simulink model "Sim_PS_DynamicOBS"  (R2018b)
settings: Solver=FixedStepAuto  StartTime=0.0  StopTime=sim_time  FixedStep=Ts  RelTol=1e-3
values from neighbouring files (symbols this model uses):
  obs1 = [x_obs1;y_obs1;r_obs1]    [Main_dynamic_obs.m]    (also in Main_static_obs.m)
  Ref = [1;1;0]    [Main_dynamic_obs.m]    (also in Main_static_obs.m)
  th0 = 0    [Main_dynamic_obs.m]    (also in Main_static_obs.m)
  Ts = 0.1    [Main_dynamic_obs.m]    (also in Main_static_obs.m)
  x0 = -1    [Main_dynamic_obs.m]    (also in Main_static_obs.m)
  x_obs2 = -0.25    [Main_dynamic_obs.m]    (also in Main_static_obs.m = 0.5)
  y0 = -1    [Main_dynamic_obs.m]    (also in Main_static_obs.m)
  y_obs2 = -0.25    [Main_dynamic_obs.m]    (also in Main_static_obs.m = 0.5)
libraries: simulink x1
settings Model: Creator=sanim  LastModifiedBy=sanim

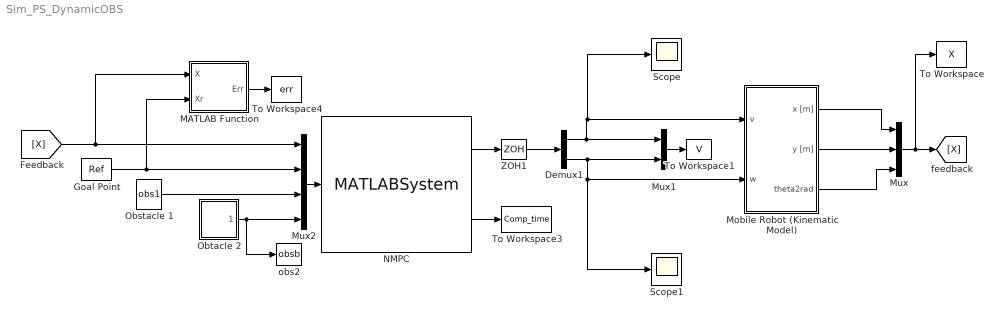
== system Sim_PS_DynamicOBS ==
  Demux1 : Demux  Outputs=2
  Goal Point : Constant  Value=Ref  SampleTime=Ts
  MATLAB Function : MATLAB Function  TreatAsAtomicUnit=on
  Mobile Robot (Kinematic Model) : Subsystem
  Mux : Mux  Inputs=3
  Mux1 : Mux  Inputs=2
  Mux2 : Mux
  NMPC : MATLABSystem  System=single_robot_obs  SimulateUsing=Interpreted execution
      mask Type: single_robot_obs
      mask Display:
      | disp('single_robot_obs');
      | port_label('input',1,'x');
      | port_label('output',1,'u');
      | port_label('output',2,'comp_time');
  Obstacle 1 : Constant  Value=obs1  SampleTime=Ts
  Obtacle 2 : Subsystem
  Scope : Scope
  Scope1 : Scope
  To Workspace : ToWorkspace  VariableName=X  SaveFormat=Structure With Time  SampleTime=Ts
  To Workspace1 : ToWorkspace  VariableName=V  SaveFormat=Structure With Time  SampleTime=Ts
  To Workspace3 : ToWorkspace  VariableName=Comp_time  SaveFormat=Structure  SampleTime=Ts
      settings: Save2DSignal=2-D array (concatenate along first dimension)
  To Workspace4 : ToWorkspace  VariableName=err  SampleTime=Ts
      settings: Save2DSignal=2-D array (concatenate along first dimension)
  ZOH1 : ZeroOrderHold  SampleTime=Ts
  obs2 : ToWorkspace  VariableName=obsb  SaveFormat=Structure  SampleTime=Ts
      settings: Save2DSignal=2-D array (concatenate along first dimension)
  wires:
  Mobile Robot (Kinematic Model)/2(y [m]) -> Mux/2
  Mux2/1 -> NMPC/1
  Demux1/1 -> Scope/1, Mobile Robot (Kinematic Model)/1(v), Mux1/1
  Mobile Robot (Kinematic Model)/3(theta2rad) -> Mux/3
  Mobile Robot (Kinematic Model)/1(x [m]) -> Mux/1
  Demux1/2 -> Scope1/1, Mobile Robot (Kinematic Model)/2(w), Mux1/2
  [X] -> MATLAB Function/1(X), Mux2/1
  Mux/1 -> To Workspace/1, [X]
  Mux1/1 -> To Workspace1/1
  NMPC/1 -> ZOH1/1
  ZOH1/1 -> Demux1/1
  Goal Point/1 -> MATLAB Function/2(Xr), Mux2/2
  NMPC/2 -> To Workspace3/1
  MATLAB Function/1(Err) -> To Workspace4/1
  Obstacle 1/1 -> Mux2/3
  Obtacle 2/1(obs2) -> obs2/1, Mux2/4

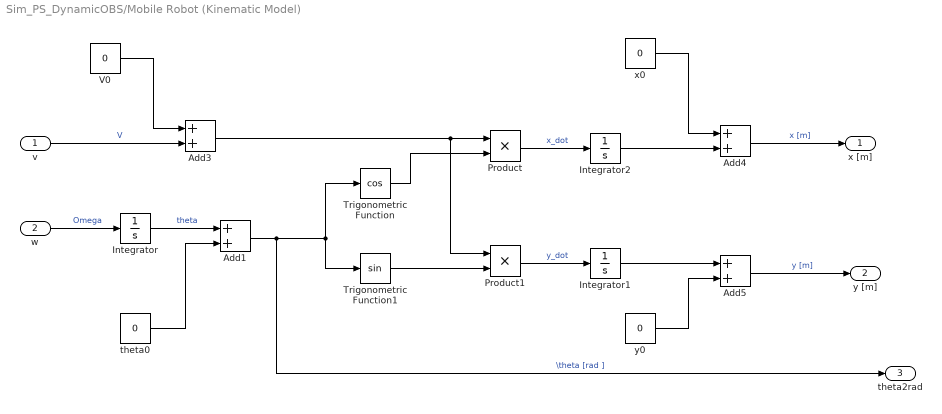
== system Sim_PS_DynamicOBS/Mobile Robot (Kinematic Model) ==
  v : Inport
  w : Inport  Port=2
  Add{1,3..5} (4 alike) : Sum
  Integrator : Integrator  InitialCondition=th0
  Integrator1 : Integrator  InitialCondition=y0
  Integrator2 : Integrator  InitialCondition=x0
  Product : Product
  Product1 : Product
  Trigonometric Function : Trigonometry  Operator=cos
  Trigonometric Function1 : Trigonometry
  "V0 " : Constant  Value=0
  theta0 : Constant  Value=0
  x0 : Constant  Value=0
  y0 : Constant  Value=0
  x [m] : Outport
  y [m] : Outport  Port=2
  theta2rad : Outport  Port=3
  wires:
  w/1 -> Integrator/1  "Omega"
  x0/1 -> Add4/1
  Product1/1 -> Integrator1/1  "y_dot"
  v/1 -> Add3/2  "V"
  theta0/1 -> Add1/2
  Trigonometric Function/1 -> Product/2
  Integrator2/1 -> Add4/2
  Add3/1 -> Product/1, Product1/1
  Add5/1 -> y [m]/1  "y [m]"
  Add4/1 -> x [m]/1  "x [m]"
  Integrator/1 -> Add1/1  "theta"
  Trigonometric Function1/1 -> Product1/2
  y0/1 -> Add5/2
  Product/1 -> Integrator2/1  "x_dot"
  Add1/1 -> Trigonometric Function/1, Trigonometric Function1/1, theta2rad/1  "\\theta [rad ]"
  "V0 "/1 -> Add3/1
  Integrator1/1 -> Add5/1

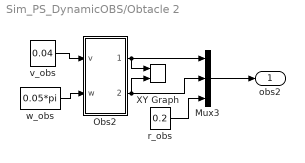
== system Sim_PS_DynamicOBS/Obtacle 2 ==
  Mux3 : Mux  Inputs=3
  Obs2 : Subsystem
  XY Graph : simulink/Sinks/XY Graph  xmin=-1  xmax=1  ymin=-1  ymax=1  st=Ts
  r_obs : Constant  Value=0.2  SampleTime=Ts
  v_obs : Constant  Value=0.04  SampleTime=Ts
  w_obs : Constant  Value=0.05*pi  SampleTime=Ts
  obs2 : Outport
  wires:
  Obs2/2(y [m]) -> Mux3/2, XY Graph/2
  w_obs/1 -> Obs2/2(w)
  Obs2/1(x [m]) -> Mux3/1, XY Graph/1
  r_obs/1 -> Mux3/3
  v_obs/1 -> Obs2/1(v)
  Mux3/1 -> obs2/1

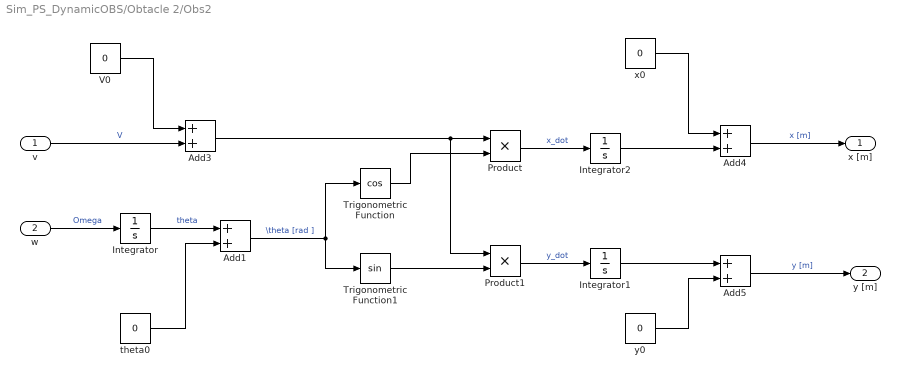
== system Sim_PS_DynamicOBS/Obtacle 2/Obs2 ==
  v : Inport
  w : Inport  Port=2
  Add{1,3..5} (4 alike) : Sum
  Integrator : Integrator  InitialCondition=-pi/4
  Integrator1 : Integrator  InitialCondition=y_obs2
  Integrator2 : Integrator  InitialCondition=x_obs2
  Product : Product
  Product1 : Product
  Trigonometric Function : Trigonometry  Operator=cos
  Trigonometric Function1 : Trigonometry
  "V0 " : Constant  Value=0
  theta0 : Constant  Value=0
  x0 : Constant  Value=0
  y0 : Constant  Value=0
  x [m] : Outport
  y [m] : Outport  Port=2
  wires:
  Integrator1/1 -> Add5/1
  "V0 "/1 -> Add3/1
  Add1/1 -> Trigonometric Function1/1, Trigonometric Function/1  "\\theta [rad ]"
  Product/1 -> Integrator2/1  "x_dot"
  y0/1 -> Add5/2
  Trigonometric Function1/1 -> Product1/2
  Integrator/1 -> Add1/1  "theta"
  Add4/1 -> x [m]/1  "x [m]"
  Add5/1 -> y [m]/1  "y [m]"
  Add3/1 -> Product1/1, Product/1
  Integrator2/1 -> Add4/2
  Trigonometric Function/1 -> Product/2
  theta0/1 -> Add1/2
  v/1 -> Add3/2  "V"
  Product1/1 -> Integrator1/1  "y_dot"
  x0/1 -> Add4/1
  w/1 -> Integrator/1  "Omega"

== matlab function Sim_PS_DynamicOBS/MATLAB Function ==
  data: X input; Err output; Xr input
function Err = fcn(X,Xr)
Ex = Xr(1) - X(1);
Ey = Xr(2) - X(2);
Et = Xr(3) - X(3);

Err = [Ex,Ey,Et];
